simulink model "inverted"  (Simulink 8.5)
settings: Solver=ode45  StartTime=0.0  StopTime=10.0  RelTol=1e-3
values from neighbouring files (symbols this model uses):
  g = 9.81    [init_pendulum.m]
  l = 0.5    [init_pendulum.m]
  m = 0.1    [init_pendulum.m]
  mc = 1.0    (= 1)    [init_pendulum.m]
  x1_0 = 0.1    [init_pendulum.m]
  x2_0 = 0.0    (= 0)    [init_pendulum.m]
libraries: fuzblock x1
settings Model: Creator=USER  LastModifiedBy=USER
settings DataIOCC: SignalLoggingSaveFormat=Dataset
settings OptimizationCC: ExpressionDepthLimit=128
settings DebuggingCC: UnderspecifiedInitializationDetection=Simplified  MergeDetectMultiDrivingBlocksExec=error  FcnCallInpInsideContextMsg=EnableAllAsError  StateNameClashWarn=none
settings GRTTargetCC: CombineOutputUpdateFcns=on  GRTInterface=off

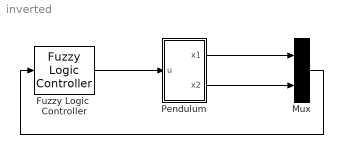
== system inverted ==
  Fuzzy Logic  Controller : fuzblock/Fuzzy Logic  Controller  fis='controller.fis'
  Mux : Mux  Inputs=2
  Pendulum : Subsystem
  wires:
  Fuzzy Logic  Controller/1 -> Pendulum/1(u)
  Pendulum/2(x2) -> Mux/2
  Pendulum/1(x1) -> Mux/1
  Mux/1 -> Fuzzy Logic  Controller/1

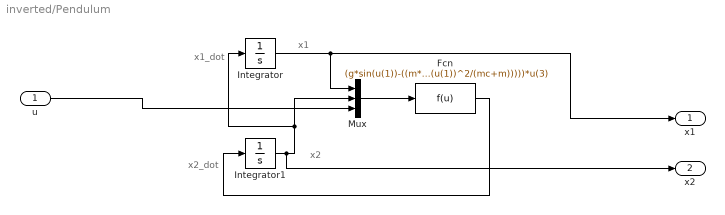
== system inverted/Pendulum ==
  note: x2
  note: x2_dot
  note: x1_dot
  note: x1
  u : Inport
  Fcn : Fcn  Expr=(g*sin(u(1))-((m*l*u(2)^2*cos(u(1))*sin(u(1))/(mc+m))))/(l*(4/3-(m*cos(u(1))^2/(mc+m))))+(cos(u(1))/(mc+m))/((l*(4/3-(m*cos(u(1))^2/(mc+m)))))*u(3)
  Integrator : Integrator  InitialCondition=x1_0
  Integrator1 : Integrator  InitialCondition=x2_0
  Mux : Mux  Inputs=3
  x1 : Outport
  x2 : Outport  Port=2
  wires:
  u/1 -> Mux/3
  Integrator1/1 -> x2/1, Mux/2, Integrator/1
  Mux/1 -> Fcn/1
  Integrator/1 -> x1/1, Mux/1
  Fcn/1 -> Integrator1/1
